simulink model "rtwdemo_slexprfold"  (Simulink 6.0)
settings: Solver=FixedStepDiscrete  StartTime=0.0  StopTime=10.0  RelTol=1e-3
PreLoadFcn:
  | rtwdemo_exprfolding_data
values from neighbouring files (symbols this model uses):
  LOWER = Simulink.Parameter    [rtwdemo_exprfolding_data.m]
  T1Break = Simulink.Parameter    [rtwdemo_exprfolding_data.m]    (also in rtwdemo_paraminline_data.m; rtwdemo_ssreuse_data.m)
  T1Data = Simulink.Parameter    [rtwdemo_exprfolding_data.m]    (also in rtwdemo_paraminline_data.m; rtwdemo_ssreuse_data.m)
  T2Data = Simulink.Parameter    [rtwdemo_exprfolding_data.m]    (also in rtwdemo_paraminline_data.m; rtwdemo_ssreuse_data.m = copy(T1Data))
  UPPER = Simulink.Parameter    [rtwdemo_exprfolding_data.m]
libraries: rtwdemowidgets x2
settings Model: CovMetricSettings=d  Creator=The MathWorks Inc.  LastModifiedBy=batserve  ExtModeAutoUpdateStatusClock=off
settings DataIOCC: SaveOutput=off  SaveTime=off  SignalLoggingName=sigsOut
settings OptimizationCC: InlineParams=on  EnforceIntegerDowncast=off  StateBitsets=on  DataBitsets=on  UseTempVars=on
settings DebuggingCC: CheckExecutionContextPreStartOutputMsg=on  CheckExecutionContextRuntimeOutputMsg=on  SignalResolutionControl=UseLocalSettings  SolverPrmCheckMsg=none
settings RTWCC: TLCOptions=-p0 -aWarnNonSaturatedBlocks=0  GenCodeOnly=on  GenerateReport=on  RTWVerbose=off  ProcessScript=grt_make_rtw_hook  LaunchReport=on
settings CodeAppCC: ForceParamTrailComments=on  PrefixModelToSubsysFcnNames=off
settings GRTTargetCC: MatFileLogging=off

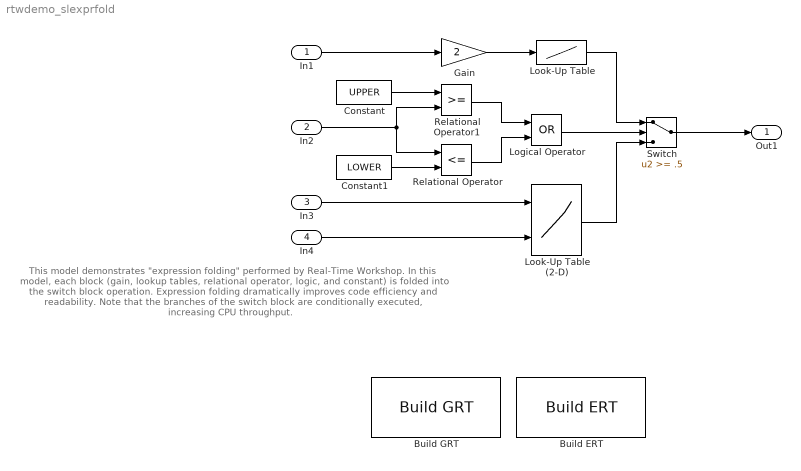
== system rtwdemo_slexprfold ==
  note: This model demonstrates "expression folding" performed by Real-Time Workshop.  In this model, each
      | block (gain, lookup tables, relational operator, logic, and constant) is folded into the switch
      | block operation.  Expression folding dramatically improves code efficiency and readability.  Note
      | that the branches of the switch block are conditionally executed, increasing CPU throughput.
  In1 : Inport  Port=1  PortDimensions=1  LatchInput=off
  In2 : Inport  Port=2  PortDimensions=1  LatchInput=off
  In3 : Inport  Port=3  PortDimensions=1  LatchInput=off
  In4 : Inport  Port=4  PortDimensions=1  LatchInput=off
  Build ERT : rtwdemowidgets/Build ERT  attrib_overrides={}
  Build GRT : rtwdemowidgets/Build GRT  attrib_overrides={}
  Constant : Constant  Value=UPPER
  Constant1 : Constant  Value=LOWER
  Gain : Gain  Gain=2  SaturateOnIntegerOverflow=on
  Logical Operator : Logic  Operator=OR
  Look-Up Table : Lookup  DialogController=Simulink.DDGSource  InputValues=T1Break  OutputValues=T1Data  SaturateOnIntegerOverflow=on
  Look-Up Table (2-D) : Lookup2D  DialogController=Simulink.DDGSource  RowIndex=T2Break  ColumnIndex=T2Break  OutputValues=T2Data  OutScaling=2^-10  InputSameDT=on
  Relational Operator : RelationalOperator  Operator=<=  InputSameDT=on
  Relational Operator1 : RelationalOperator  InputSameDT=on
  Switch : Switch  Threshold=.5  SaturateOnIntegerOverflow=on  InputSameDT=on
  Out1 : Outport
  wires:
  Relational Operator1/1 -> Logical Operator/1
  Relational Operator/1 -> Logical Operator/2
  Logical Operator/1 -> Switch/2
  Constant1/1 -> Relational Operator/2
  In1/1 -> Gain/1
  Look-Up Table/1 -> Switch/1
  Switch/1 -> Out1/1
  Gain/1 -> Look-Up Table/1
  Look-Up Table (2-D)/1 -> Switch/3
  Constant/1 -> Relational Operator1/1
  In2/1 -> Relational Operator1/2, Relational Operator/1
  In3/1 -> Look-Up Table (2-D)/1
  In4/1 -> Look-Up Table (2-D)/2
